simulink model "VAB_non_linear"  (R2019b)
settings: Solver=FixedStepAuto  StartTime=0.0  StopTime=t_end  FixedStep=Ts  RelTol=1e-3
values from neighbouring files (symbols this model uses):
  alpha = fliplr(poly(A))    [Calcola_T_alpha.m]    (also in fdt_vab_lineare.m = alfa)
  K = [-0.00227126037234 -0.0278341382787 -28.1396904229 -7.70218039791]    [K.mat]
undefined symbols (not defined in the file or in its folder): control_on, phi_secondo, theta_iniziale, theta_secondo
settings Model: Creator=miche  LastModifiedBy=AndreaCalegari

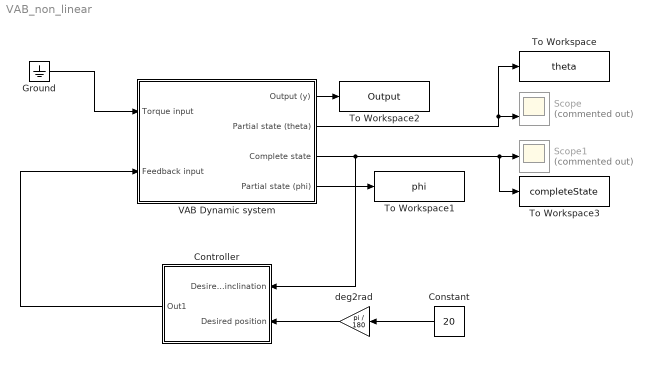
== system VAB_non_linear ==
  Constant : Constant  Value=20
  Controller : Subsystem
  Ground : Ground
  Scope : Scope  Commented=on  NumInputPorts=2
  Scope1 : Scope  Commented=on
  To Workspace : ToWorkspace  VariableName=theta  SampleTime=-1
  To Workspace1 : ToWorkspace  VariableName=phi  SampleTime=-1
  To Workspace2 : ToWorkspace  VariableName=Output  SampleTime=-1
  To Workspace3 : ToWorkspace  VariableName=completeState  SampleTime=-1
  VAB Dynamic system : Subsystem
  deg2rad : Gain  Gain=pi / 180
  wires:
  VAB Dynamic system/3("Complete state ") -> Controller/1(Desired inclination), Scope1/1, To Workspace3/1
  VAB Dynamic system/2(Partial state (theta)) -> To Workspace/1, Scope/2
  VAB Dynamic system/1(Output (y)) -> To Workspace2/1
  Controller/1(Out1) -> VAB Dynamic system/2(Feedback input)
  VAB Dynamic system/4(Partial state (phi)) -> To Workspace1/1
  Constant/1 -> deg2rad/1
  deg2rad/1 -> Controller/2("Desired position ")
  Ground/1 -> VAB Dynamic system/1(Torque input)

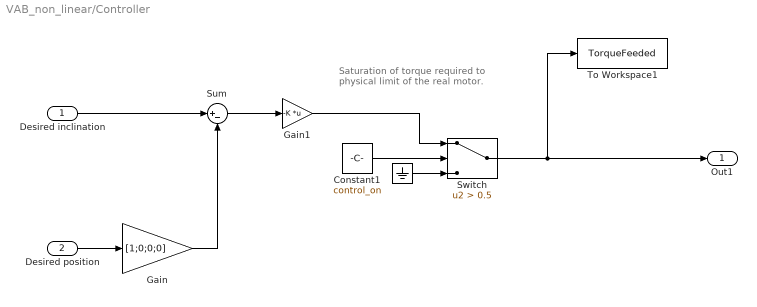
== system VAB_non_linear/Controller ==
  note: Saturation of torque required
      | to physical limit of the real motor.
  Desired inclination : Inport
  "Desired position " : Inport  Port=2
  " " : Ground
  Constant1 : Constant  Value=control_on
  Gain : Gain  Gain=[1;0;0;0]
  Gain1 : Gain  Gain=-K  Multiplication=Matrix(K*u)
  Sum : Sum  Inputs=|+-
  Switch : Switch  Criteria=u2 > Threshold  Threshold=0.5
  To Workspace1 : ToWorkspace  VariableName=TorqueFeeded  SampleTime=-1
  Out1 : Outport
  wires:
  Constant1/1 -> Switch/2
  " "/1 -> Switch/3
  Sum/1 -> Gain1/1
  Desired inclination/1 -> Sum/1
  Gain/1 -> Sum/2
  "Desired position "/1 -> Gain/1
  Gain1/1 -> Switch/1
  Switch/1 -> Out1/1, To Workspace1/1

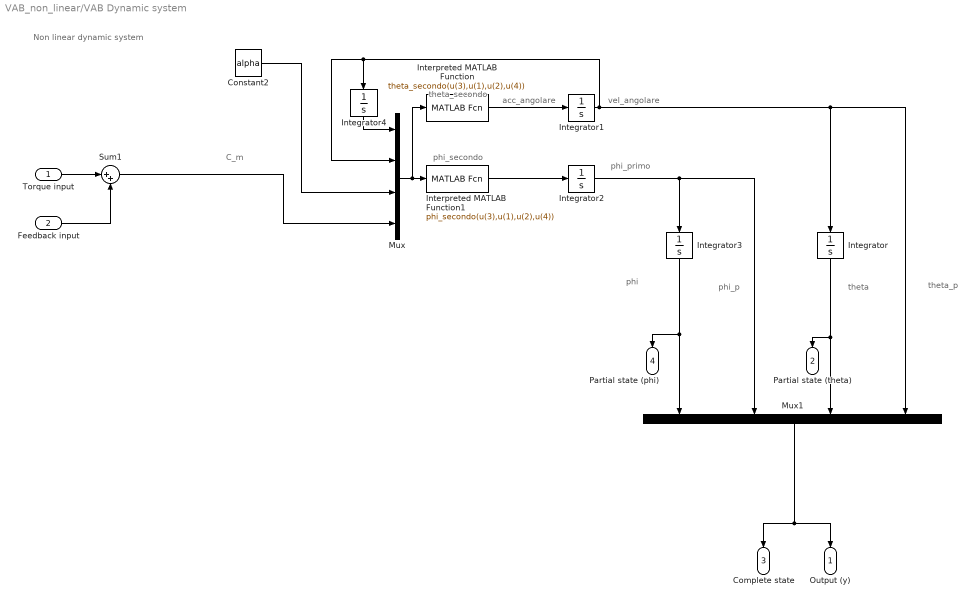
== system VAB_non_linear/VAB Dynamic system ==
  note: Non linear dynamic system
  note: phi_primo
  note: phi
  note: theta_p
  note: theta
  note: phi_p
  note: phi_secondo
  note: C_m
  note: acc_angolare
  note: theta_secondo
  note: vel_angolare
  Torque input : Inport
  Feedback input : Inport  Port=2
  Constant2 : Constant  Value=alpha
  Integrator : Integrator  InitialCondition=theta_iniziale
  Integrator1 : Integrator  UpperSaturationLimit=100  LowerSaturationLimit=-100
  Integrator2 : Integrator
  Integrator3 : Integrator
  Integrator4 : Integrator  InitialCondition=theta_iniziale
  Interpreted MATLAB Function : MATLABFcn  MATLABFcn=theta_secondo(u(3),u(1),u(2),u(4))  OutputDimensions=1
  Interpreted MATLAB Function1 : MATLABFcn  MATLABFcn=phi_secondo(u(3),u(1),u(2),u(4))
  Mux : Mux
  Mux1 : Mux
  Sum1 : Sum  Inputs=|++
  Output (y) : Outport
  Partial state (theta) : Outport  Port=2
  "Complete state " : Outport  Port=3
  Partial state (phi) : Outport  Port=4
  wires:
  Feedback input/1 -> Sum1/2
  Torque input/1 -> Sum1/1
  Integrator3/1 -> Partial state (phi)/1, Mux1/1
  Constant2/1 -> Mux/3
  Sum1/1 -> Mux/4
  Integrator4/1 -> Mux/1
  Interpreted MATLAB Function1/1 -> Integrator2/1
  Integrator2/1 -> Mux1/2, Integrator3/1
  Mux/1 -> Interpreted MATLAB Function/1, Interpreted MATLAB Function1/1
  Integrator1/1 -> Integrator4/1, Mux/2, Mux1/4, Integrator/1
  Integrator/1 -> Partial state (theta)/1, Mux1/3
  Interpreted MATLAB Function/1 -> Integrator1/1
  Mux1/1 -> Output (y)/1, "Complete state "/1
